simulink model "Calculator"  (R2021a)
settings: Solver=FixedStepDiscrete  StartTime=0.0  StopTime=10.0  RelTol=1e-3  EnableMultiTasking=on
settings Model: Creator=top one  LastModifiedBy=top one
settings DataIOCC: ReturnWorkspaceOutputs=off
settings OptimizationCC: DefaultParameterBehavior=Inlined  InlineInvariantSignals=on  EnableMemcpy=off  LifeSpan=1  EfficientTunableParamExpr=on
settings DebuggingCC: UnderspecifiedInitializationDetection=Classic  MergeDetectMultiDrivingBlocksExec=none  SFMachineParentedDataDiag=warning  ArithmeticOperatorsInVariantConditions=warning
settings ModelReferenceCC: PropagateSignalLabelsOutOfModel=off
settings SFSimCC: MATLABDynamicMemAlloc=off  CustomCodeUndefinedFunction=UseInterfaceOnly
settings RTWCC: SystemTargetFile=ert.tlc  GenCodeOnly=on  TemplateMakefile=ert_default_tmf  GenerateReport=on  IncludeHyperlinkInReport=on  LaunchReport=on  GenerateTraceInfo=on  GenerateTraceReport=on  GenerateTraceReportSl=on  GenerateTraceReportSf=on  GenerateTraceReportEml=on
settings CodeAppCC: ForceParamTrailComments=on  IgnoreCustomStorageClasses=off  OperatorAnnotations=on  SimulinkDataObjDesc=on  SFDataObjDesc=on  MATLABFcnDesc=on  InsertBlockDesc=on  StateflowObjectComments=on  MATLABSourceComments=on
settings ERTTargetCC: MultiwordLength=2048  GenerateSampleERTMain=on  InlinedParameterPlacement=NonHierarchical  ERTCustomFileTemplate=example_file_process.tlc

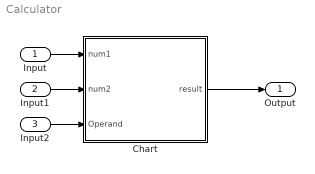
== system Calculator ==
  Input : Inport
  Input1 : Inport  Port=2
  Input2 : Inport  Port=3
  Chart : Stateflow chart  TreatAsAtomicUnit=on
  Output : Outport
  wires:
  Chart/1(result) -> Output/1
  Input/1 -> Chart/1(num1)
  Input1/1 -> Chart/2(num2)
  Input2/1 -> Chart/3(Operand)

== stateflow chart Calculator/Chart ==
  state add(n1,n2) [function]
    (default) -> (junction 53) : {result=n1+n2;}
  note: Do not put any code along
      | the transitions that run
      | down the right side!
  state sub(n1,n2) [function]
    (default) -> (junction 58) : {result=n1-n2;}
  state mul(n1,n2) [function]
    (default) -> (junction 63) : {result=n1*n2;}
  state div(n1,n2) [function]
    (default) -> (junction 71) : {result=n1/n2;}
  (default) -> (junction 25) : % Calculator
  (junction 25) -> (junction 26) [order 1] : [Operand == 1]
  (junction 25) -> (junction 29) [order 2]
  (junction 26) -> (junction 27) : {add(num1,num2);}
  (junction 27) -> (junction 28)
  (junction 28) -> (junction 32)
  (junction 29) -> (junction 30) [order 1] : [Operand == 2]
  (junction 29) -> (junction 33) [order 2]
  (junction 30) -> (junction 31) : {sub(num1,num2);}
  (junction 31) -> (junction 32)
  (junction 32) -> (junction 36)
  (junction 33) -> (junction 34) [order 1] : [Operand == 3]
  (junction 33) -> (junction 37) [order 2]
  (junction 34) -> (junction 35) : {mul(num1,num2);}
  (junction 35) -> (junction 36)
  (junction 36) -> (junction 40)
  (junction 37) -> (junction 38) [order 1] : [Operand == 4]
  (junction 37) -> (junction 41) [order 2]
  (junction 38) -> (junction 39) : {div(num1,num2);}
  (junction 39) -> (junction 40)
  (junction 40) -> (junction 42)
  (junction 42) -> (junction 41)
  (junction 41) -> (junction 43)
  data: n1 function_input; n2 function_input; n1 function_input; n2 function_input; n1 function_input; n2 function_input; n1 function_input; n2 function_input; num1 input; num2 input; Operand input; result output
